simulink model "cassandra_model"  (R2025b)
settings: Solver=FixedStepAuto  StartTime=0.0  StopTime=1800  FixedStep=0.1  RelTol=1e-3
model workspace (MAT data in the model file):
  D_normal = 200
  D_total = 500
  T_outage = 600
  base_latency = 0.005
  read_rate = 5000
  read_timeout = 0.5
  repair_cost = 3
  replay_throttle = 128
  write_rate = 10000
settings Model: Creator=aalpar  LastModifiedBy=aalpar

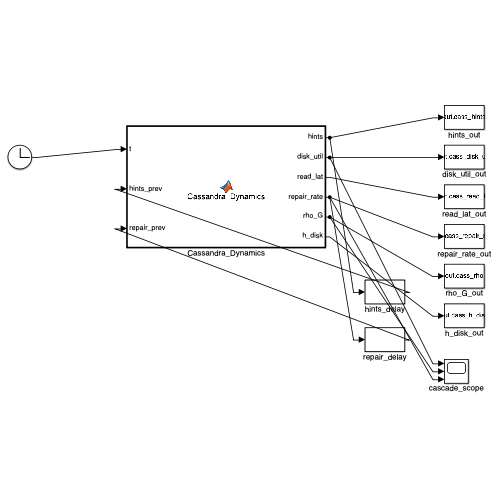
[thumbnail: Simulink's stored preview of the top-level diagram]
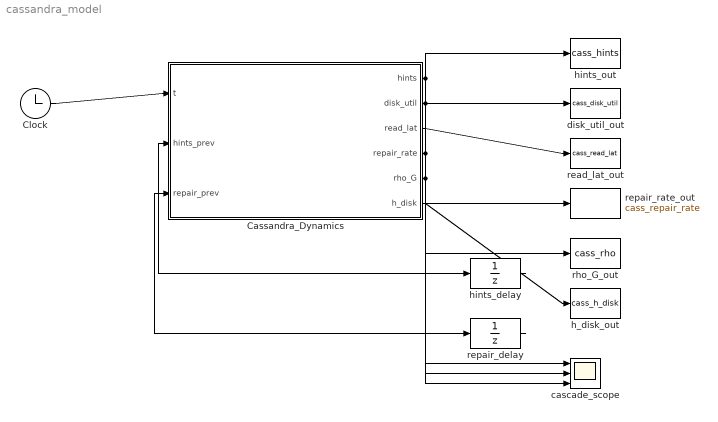
== system cassandra_model ==
  Cassandra_Dynamics : MATLAB Function  TreatAsAtomicUnit=on
  Clock : Clock
  cascade_scope : Scope  NumInputPorts=3
  disk_util_out : ToWorkspace  VariableName=cass_disk_util  SaveFormat=Timeseries  SampleTime=-1
  h_disk_out : ToWorkspace  VariableName=cass_h_disk  SaveFormat=Timeseries  SampleTime=-1
  hints_delay : UnitDelay  SampleTime=0.1  HasFrameUpgradeWarning=on
  hints_out : ToWorkspace  VariableName=cass_hints  SaveFormat=Timeseries  SampleTime=-1
  read_lat_out : ToWorkspace  VariableName=cass_read_lat  SaveFormat=Timeseries  SampleTime=-1
  repair_delay : UnitDelay  SampleTime=0.1  HasFrameUpgradeWarning=on
  repair_rate_out : ToWorkspace  VariableName=cass_repair_rate  SaveFormat=Timeseries  SampleTime=-1
  rho_G_out : ToWorkspace  VariableName=cass_rho  SaveFormat=Timeseries  SampleTime=-1
  wires:
  Clock/1 -> Cassandra_Dynamics/1(t)
  hints_delay/1 -> Cassandra_Dynamics/2(hints_prev)
  repair_delay/1 -> Cassandra_Dynamics/3(repair_prev)
  Cassandra_Dynamics/1(hints) -> hints_out/1, hints_delay/1
  Cassandra_Dynamics/2(disk_util) -> disk_util_out/1, cascade_scope/1
  Cassandra_Dynamics/3(read_lat) -> read_lat_out/1
  Cassandra_Dynamics/4(repair_rate) -> repair_rate_out/1, repair_delay/1, cascade_scope/3
  Cassandra_Dynamics/5(rho_G) -> rho_G_out/1, cascade_scope/2
  Cassandra_Dynamics/6(h_disk) -> h_disk_out/1

== matlab function cassandra_model/Cassandra_Dynamics ==
  data: t input; hints output; hints_prev input; repair_prev input; disk_util output; read_lat output; repair_rate output; rho_G output; h_disk output
function [hints, disk_util, read_lat, repair_rate, rho_G, h_disk] = Cassandra_Dynamics(t, hints_prev, repair_prev)
persistent accumulated_hints
if isempty(accumulated_hints), accumulated_hints = 0; end

write_rate = 10000; read_rate = 5000; T_outage = 600;
replay_throttle = 128;
D_total = 500; D_normal = 200;
base_latency = 0.005; read_timeout = 0.5;
repair_cost = 3;

% Phase 1: Outage — hints accumulate
if t < T_outage
    accumulated_hints = accumulated_hints + write_rate * 0.1;  % dt=0.1
    replay_iops = 0;
else
    % Phase 2: Replay
    replay_iops = min(replay_throttle, accumulated_hints / 0.1);
    accumulated_hints = max(0, accumulated_hints - replay_iops * 0.1);
end
hints = accumulated_hints;

% Disk utilization
total_iops = D_normal + replay_iops + repair_prev * repair_cost;
disk_util = min(total_iops / D_total, 0.999);

% Read latency (M/M/1)
read_lat = base_latency / (1 - disk_util);

% Read repair rate
if read_lat > read_timeout
    timeout_frac = min(1, (read_lat - read_timeout) / read_lat);
else
    timeout_frac = 0;
end
repair_rate = read_rate * timeout_frac;

% Headroom
h_disk = D_total - total_iops;

% Gain matrix (instantaneous)
if D_total > 0
    g_dd = repair_cost * repair_rate / D_total;
else
    g_dd = 0;
end
G = [g_dd, 0.1; 0.01*repair_rate, 0.1];
rho_G = max(abs(eig(G)));
